simulink subsystem "bus_from_vector"  (R2024a)
settings: Solver=VariableStepAuto  StartTime=0.0  StopTime=10.0  RelTol=1e-3
model mask{bus=0, BusTemplate=0}
  mask prompts: BusTemplate "Bus Template"
settings Model: Creator=Friedrich Tuttas  LastModifiedBy=Friedrich Tuttas

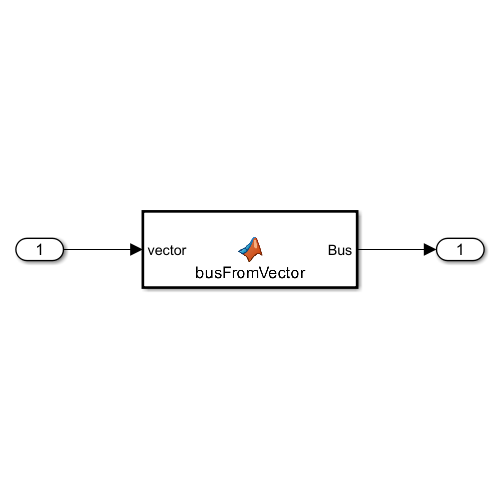
[thumbnail: Simulink's stored preview of the top-level diagram]
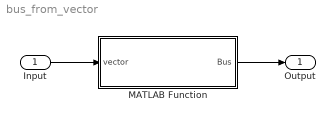
== system bus_from_vector ==
  Input : Inport
  MATLAB Function : MATLAB Function  TreatAsAtomicUnit=on
  Output : Outport
  wires:
  MATLAB Function/1(Bus) -> Output/1
  Input/1 -> MATLAB Function/1(vector)

== matlab function bus_from_vector/MATLAB Function ==
  data: vector input; Bus output Bus: bus; BusTemplate parameter
function Bus = busFromVector(vector, BusTemplate)

Bus = BusTemplate;

[Bus, ~] = populateNumericStructureFromVector(Bus, vector);

end
